simulink model "lab4_2"  (R2018a)
settings: Solver=ode45  StartTime=0.0  StopTime=15  MaxStep=0.001  RelTol=1e-3
values from neighbouring files (symbols this model uses):
  A = Rs*(Ps^(-1))    [modele04.m]
  B = [ 0; 0]    [modele04.m]
  C = [ 1 0 ; 0 1 ]    [modele04.m]
  D = [ 0 ; 0 ]    [modele04.m]
settings Model: Creator=Koala  LastModifiedBy=Koala

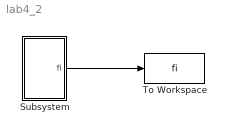
== system lab4_2 ==
  Subsystem : Subsystem  mask{m=2, k=2, g=9.81, l=1, fi0=90}
  To Workspace : ToWorkspace  VariableName=fi  SampleTime=-1
  wires:
  Subsystem/1(fi) -> To Workspace/1

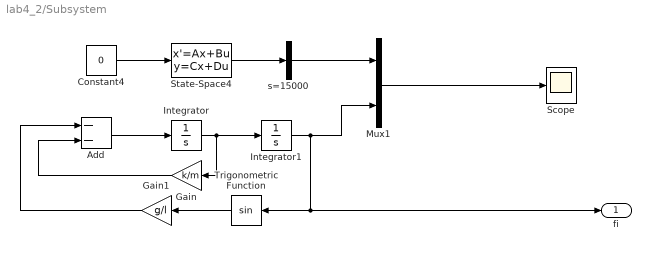
== system lab4_2/Subsystem ==
  Add : Sum  Inputs=--
  Constant4 : Constant  Value=0
  Gain : Gain  Gain=k/m
  Gain1 : Gain  Gain=g/l
  Integrator : Integrator
  Integrator1 : Integrator  InitialCondition=fi0*pi/180
  Mux1 : Mux  Inputs=2
  Scope : Scope
  State-Space4 : StateSpace  A=A  B=B  C=C  D=D  InitialCondition=[pi/2 0]
  Trigonometric Function : Trigonometry
  s=15000 : Demux  Outputs=1
  fi : Outport
  wires:
  Gain/1 -> Add/2
  Add/1 -> Integrator/1
  Integrator/1 -> Gain/1, Integrator1/1
  Trigonometric Function/1 -> Gain1/1
  Gain1/1 -> Add/1
  Mux1/1 -> Scope/1
  Integrator1/1 -> Mux1/2, fi/1, Trigonometric Function/1
  s=15000/1 -> Mux1/1
  Constant4/1 -> State-Space4/1
  State-Space4/1 -> s=15000/1
